simulink model "DuoCopter1AGRESSIVE"  (R2015b)
settings: Solver=FixedStepAuto  StartTime=0.0  StopTime=100  FixedStep=.01  MaxStep=10  RelTol=1e-3
values from neighbouring files (symbols this model uses):
  AoAMax = 18    [MainDataFile.m]
  RodMass = 1505    [MainDataFile.m]
  s = saveObjectImpl@matlab.System(obj)    [moving_average.m]
undefined symbols (not defined in the file or in its folder): X, Y, Z
libraries: sm_lib x35, Library_Octocopter x19, nesl_utility x17, simulink x3, aerolibfltsims x2
(part 1 of 2)
settings Model: Creator=John  LastModifiedBy=hielke
settings SolverCC: AutoInsertRateTranBlk=on
settings DataIOCC: SaveFormat=Array
settings OptimizationCC: OptimizeBlockIOStorage=off  BufferReuse=off  GlobalBufferReuse=off  ExpressionFolding=off  LocalBlockOutputs=off
settings DebuggingCC: UnderspecifiedInitializationDetection=Classic  MergeDetectMultiDrivingBlocksExec=none  SolverPrmCheckMsg=warning
settings HardwareCC: ProdBitPerLong=64  ProdHWDeviceType=Intel->x86-64 (Linux 64)
settings GRTTargetCC: GeneratePreprocessorConditionals=Disable all
settings ConfigComp: CovModelRefEnable=Off

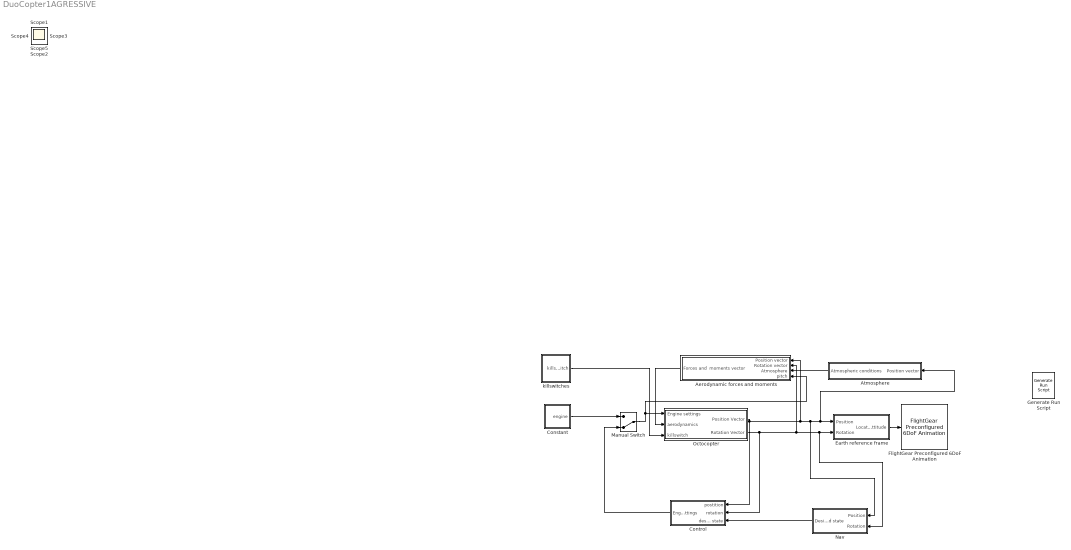
== system DuoCopter1AGRESSIVE ==
  Aerodynamic forces and moments : Subsystem
  Atmosphere : Subsystem
  Constant : Subsystem
  Control : Subsystem
  Earth reference frame : Subsystem
  FlightGear Preconfigured 6DoF Animation : aerolibfltsims/FlightGear Preconfigured 6DoF Animation  xFlightGearVersion=v3.4  DestinationIpAddress=127.0.0.1  DestinationPort=5502  SampleTime=-1
  Generate Run Script : aerolibfltsims/Generate Run Script  OutputFileName=runfg.sh  FlightGearBaseDirectory=/usr/share/games/flightgear  GeometryModelName=HL20  DestinationPort=5502  OriginAddress=127.0.0.1  OriginPort=5505  LocalAddress=127.0.0.1  AirportId=KSFO  RunwayId=10L  InitialAltitude=7224  InitialHeading=113  OffsetDistance=4.72  OffsetAzimuth=0  GenerateFile=off  Architecture=Linux  dataFlow=Send
  Manual Switch : ManualSwitch  CurrentSetting=0
  Nav : Subsystem
  Octocopter : Subsystem  SystemSampleTime=0.01
      settings: MinAlgLoopOccurrences=on
  killswitches : Subsystem
  Scope{,1..5} (6 alike) : Scope
  wires:
  Octocopter/2(Rotation Vector) -> Control/2(rotation), Aerodynamic forces and moments/2(Rotation vector), Nav/2(Rotation), Earth reference frame/2(Rotation)
  Octocopter/1(Position Vector) -> Control/1(postition), Aerodynamic forces and moments/1(Position vector), Nav/1(Position), Atmosphere/1(Position vector), Earth reference frame/1(Position)
  Nav/1(Desired state) -> Control/3(desired state)
  Earth reference frame/1(Location and attitude) -> FlightGear Preconfigured 6DoF Animation/1
  Control/1(Engine settings) -> Manual Switch/2
  Constant/1(engine) -> Manual Switch/1
  Manual Switch/1 -> Aerodynamic forces and moments/4(pitch), Octocopter/1(Engine settings)
  Aerodynamic forces and moments/1(Forces and  moments vector) -> Octocopter/2(aerodynamics)
  Atmosphere/1(Atmospheric conditions) -> Aerodynamic forces and moments/3(Atmosphere)
  killswitches/1(killswitch) -> Octocopter/3("killswitch ")

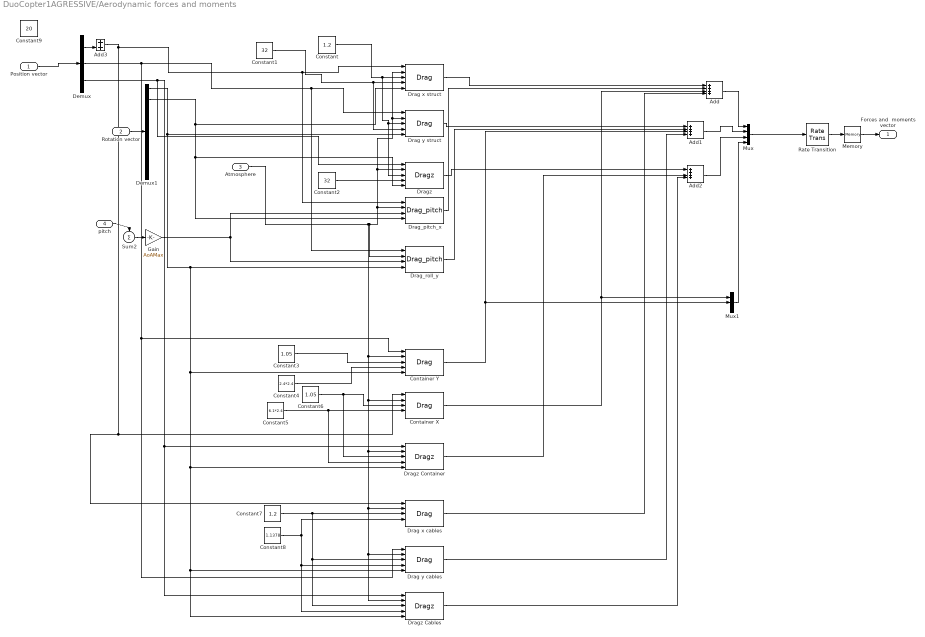
== system DuoCopter1AGRESSIVE/Aerodynamic forces and moments ==
  Position vector : Inport
  Rotation vector : Inport  Port=2
  Atmosphere : Inport  Port=3
  pitch : Inport  Port=4
  Add : Sum  Inputs=++++
  Add1 : Sum  Inputs=++++
  Add2 : Sum  Inputs=++++
  Add3 : Sum
  Constant : Constant  Value=1.2  SampleTime=1
  Constant1 : Constant  Value=32  SampleTime=1
  Constant2 : Constant  Value=32  SampleTime=1
  Constant3 : Constant  Value=1.05  SampleTime=1
  Constant4 : Constant  Value=2.4*2.4  SampleTime=1
  Constant5 : Constant  Value=6.1*2.4  SampleTime=1
  Constant6 : Constant  Value=1.05  SampleTime=1
  Constant7 : Constant  Value=1.2  SampleTime=1
  Constant8 : Constant  Value=1.1378  SampleTime=1
  Constant9 : Constant  Value=20
  Container X : Library_Octocopter/Drag
  Container Y : Library_Octocopter/Drag
  Demux : Demux  Outputs=9
  Demux1 : Demux  Outputs=9
  Drag x cables : Library_Octocopter/Drag
  Drag x struct : Library_Octocopter/Drag
  Drag y cables : Library_Octocopter/Drag
  Drag y struct : Library_Octocopter/Drag
  Drag_pitch_x : Library_Octocopter/Drag_pitch
  Drag_roll_y : Library_Octocopter/Drag_pitch
  "Dragz " : Library_Octocopter/Dragz 
  Dragz Cables : Library_Octocopter/Dragz 
  Dragz Container : Library_Octocopter/Dragz 
  Gain : Gain  Gain=AoAMax
  Memory : Memory  InheritSampleTime=on  LinearizeMemory=on  LinearizeAsDelay=on
  Mux : Mux
  Mux1 : Mux  Inputs=3
  Rate Transition : RateTransition  OutPortSampleTimeOpt=Inherit
  Sum2 : Sum  Inputs=+|
  Forces and  moments vector : Outport
  wires:
  Position vector/1 -> Demux/1
  Demux/5 -> Drag y cables/1, Container Y/1, Drag_roll_y/1, Drag y struct/1
  Atmosphere/1 -> Container X/2, Dragz Container/2, Drag x cables/2, Dragz Cables/2, Drag y cables/2, Container Y/2, Drag_roll_y/2, "Dragz "/2, Drag x struct/2, Drag y struct/2, Drag_pitch_x/2
  Constant/1 -> Drag x struct/3, "Dragz "/3, Drag y struct/3
  Constant1/1 -> Drag y struct/4, Drag x struct/4
  Constant2/1 -> "Dragz "/4
  Add3/1 -> Drag_pitch_x/1, Drag x struct/1, Drag x cables/1, Container X/1
  Demux/8 -> Dragz Cables/1, Dragz Container/1, "Dragz "/1
  Rotation vector/1 -> Demux1/1
  Demux1/1 -> Drag y struct/5, Dragz Cables/5, Drag y cables/5, Dragz Container/5, Container Y/5, Drag_roll_y/4
  Demux1/2 -> Drag x struct/5, "Dragz "/5, Drag_pitch_x/4
  Add1/1 -> Mux/2
  Drag x struct/1 -> Add/1
  Add/1 -> Mux/1
  Mux/1 -> Rate Transition/1
  pitch/1 -> Sum2/1
  Sum2/1 -> Gain/1
  Gain/1 -> Drag_roll_y/3, Drag_pitch_x/3
  Drag y struct/1 -> Add1/1
  Drag_roll_y/1 -> Add1/2
  Drag_pitch_x/1 -> Add/2
  Mux1/1 -> Mux/4
  Rate Transition/1 -> Memory/1
  Memory/1 -> Forces and  moments vector/1
  Constant3/1 -> Container Y/3
  Constant4/1 -> Container Y/4
  Constant5/1 -> Dragz Container/4, Container X/4
  Constant6/1 -> Dragz Container/3, Container X/3
  Constant7/1 -> Drag x cables/3, Dragz Cables/3, Drag y cables/3
  Constant8/1 -> Drag x cables/4, Dragz Cables/4, Drag y cables/4
  Container X/1 -> Add/3, Mux1/1
  Container Y/1 -> Mux1/2, Add1/3
  Drag x cables/1 -> Add/4
  Drag y cables/1 -> Add1/4
  "Dragz "/1 -> Add2/1
  Add2/1 -> Mux/3
  Dragz Container/1 -> Add2/3
  Dragz Cables/1 -> Add2/4
  Demux/2 -> Add3/2

== system DuoCopter1AGRESSIVE/Atmosphere ==
  Position vector : Inport
  Demux : Demux  Outputs=9
  MATLAB Function : MATLAB Function  TreatAsAtomicUnit=on  SystemSampleTime=10
      settings: MinAlgLoopOccurrences=on
  Rate Transition : RateTransition  X0=1.225  OutPortSampleTime=10
  Rate Transition1 : RateTransition  X0=1.225
  Atmospheric conditions : Outport
  wires:
  Position vector/1 -> Rate Transition/1
  Demux/3 -> MATLAB Function/1(u)
  MATLAB Function/1(y) -> Rate Transition1/1
  Rate Transition/1 -> Demux/1
  Rate Transition1/1 -> Atmospheric conditions/1

== system DuoCopter1AGRESSIVE/Constant ==
  Constant7 : Constant  Value=0.835
  Mux : Mux  Inputs=8
  engine : Outport
  wires:
  Mux/1 -> engine/1
  Constant7/1 -> Mux/1, Mux/2, Mux/3, Mux/4, Mux/5, Mux/6, Mux/7, Mux/8

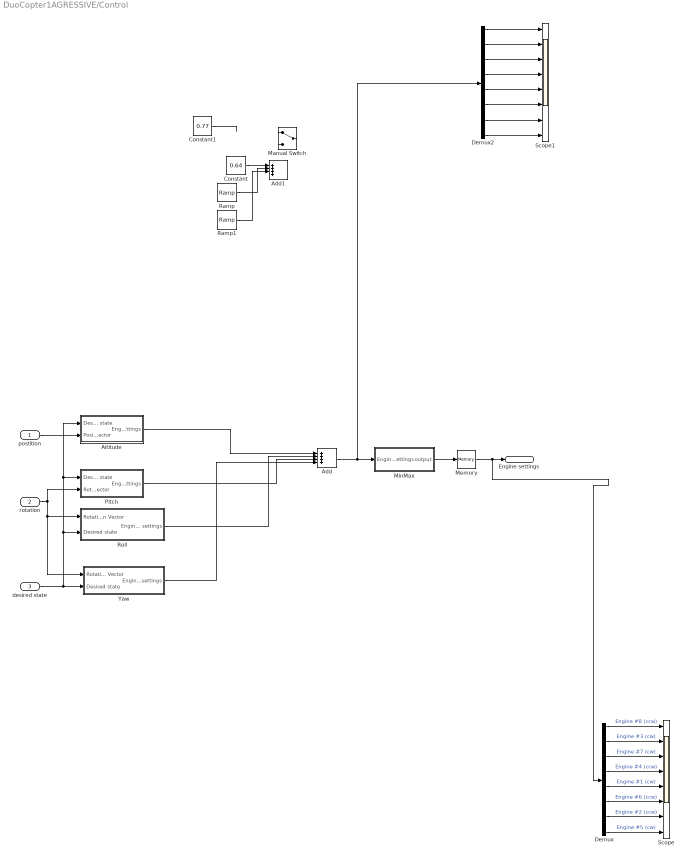
== system DuoCopter1AGRESSIVE/Control ==
  postition : Inport
  rotation : Inport  Port=2
  desired state : Inport  Port=3
  Add : Sum  Inputs=++++
  Add1 : Sum  Inputs=++++
  Altitude : Subsystem
  Constant : Constant  Value=0.64
  Constant1 : Constant  Value=0.77
  Demux : Demux  Outputs=8
  Demux2 : Demux  Outputs=8
  Manual Switch : ManualSwitch
  Memory : Memory  X0=0.84  InheritSampleTime=on  LinearizeMemory=on  LinearizeAsDelay=on
  MinMax : Subsystem
  Pitch : Subsystem
  Ramp : simulink/Sources/Ramp  slope=.014  start=20  X0=0
  Ramp1 : simulink/Sources/Ramp  slope=-.014  start=42  X0=0
  Roll : Subsystem
  Scope : Scope  NumInputPorts=8
  Scope1 : Scope  NumInputPorts=8
  Yaw : Subsystem
  Engine settings : Outport
  wires:
  Roll/1(Engine settings) -> Add/2
  Pitch/1(Engine settings) -> Add/3
  Yaw/1(Engine settings) -> Add/4
  Demux/1 -> Scope/1  "Engine #8 (ccw)"
  Demux/2 -> Scope/2  "Engine #3 (cw)"
  Demux/3 -> Scope/3  "Engine #7 (cw)"
  Demux/4 -> Scope/4  "Engine #4 (ccw)"
  Demux/5 -> Scope/5  "Engine #1 (cw)"
  Demux/6 -> Scope/6  "Engine #6 (ccw)"
  Demux/7 -> Scope/7  "Engine #2 (ccw)"
  Demux/8 -> Scope/8  "Engine #5 (cw)"
  Demux2/1 -> Scope1/1
  Demux2/2 -> Scope1/2
  Demux2/3 -> Scope1/3
  Demux2/4 -> Scope1/4
  Demux2/5 -> Scope1/5
  Demux2/6 -> Scope1/6
  Demux2/7 -> Scope1/7
  Demux2/8 -> Scope1/8
  Memory/1 -> Demux/1, Engine settings/1
  Add/1 -> Demux2/1, MinMax/1(Engine settings)
  rotation/1 -> Yaw/1(Rotation Vector), Roll/1(Rotation Vector), Pitch/2(Rotation Vector)
  desired state/1 -> Yaw/2(Desired state), Altitude/1(Desired state), Pitch/1(Desired state), Roll/2(Desired state)
  postition/1 -> Altitude/2(Position Vector)
  MinMax/1(output) -> Memory/1
  Constant/1 -> Add1/1
  Constant1/1 -> ?
  Ramp/1 -> Add1/2
  Ramp1/1 -> Add1/3
  Altitude/1(Engine settings) -> Add/1

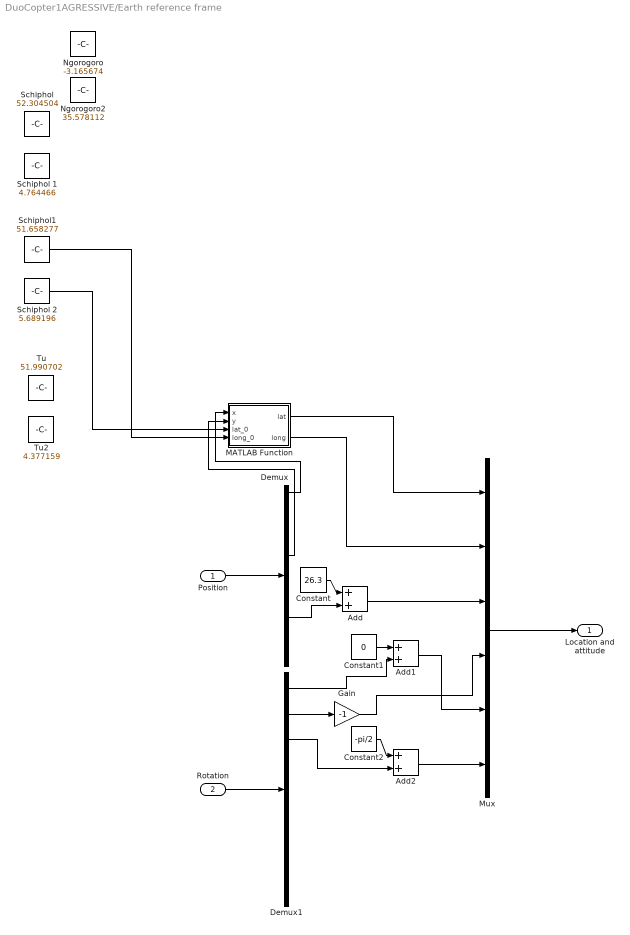
== system DuoCopter1AGRESSIVE/Earth reference frame ==
  Position : Inport
  Rotation : Inport  Port=2
  Add : Sum
  Add1 : Sum
  Add2 : Sum
  Constant : Constant  Value=26.3
  Constant1 : Constant  Value=0
  Constant2 : Constant  Value=-pi/2
  Demux : Demux  Outputs=9
  Demux1 : Demux  Outputs=9
  Gain : Gain  Gain=-1
  MATLAB Function : MATLAB Function  TreatAsAtomicUnit=on
  Mux : Mux  Inputs=6
  Ngorogoro : Constant  Value=-3.165674
  Ngorogoro2 : Constant  Value=35.578112
  Schiphol : Constant  Value=52.304504
  Schiphol 1 : Constant  Value=4.764466
  Schiphol 2 : Constant  Value=5.689196
  Schiphol1 : Constant  Value=51.658277
  Tu : Constant  Value=51.990702
  "Tu2 " : Constant  Value=4.377159
  Location and attitude : Outport
  wires:
  Position/1 -> Demux/1
  Rotation/1 -> Demux1/1
  Demux1/2 -> Gain/1
  Mux/1 -> Location and attitude/1
  Demux/7 -> Add/2
  Constant/1 -> Add/1
  Add/1 -> Mux/3
  Demux/1 -> MATLAB Function/1(x)
  Demux/4 -> MATLAB Function/2(y)
  MATLAB Function/1(lat) -> Mux/1
  MATLAB Function/2(long) -> Mux/2
  Demux1/1 -> Add1/2
  Constant1/1 -> Add1/1
  Add1/1 -> Mux/5
  Schiphol1/1 -> MATLAB Function/4(long_0)
  Schiphol 2/1 -> MATLAB Function/3(lat_0)
  Demux1/3 -> Add2/2
  Constant2/1 -> Add2/1
  Add2/1 -> Mux/6
  Gain/1 -> Mux/4

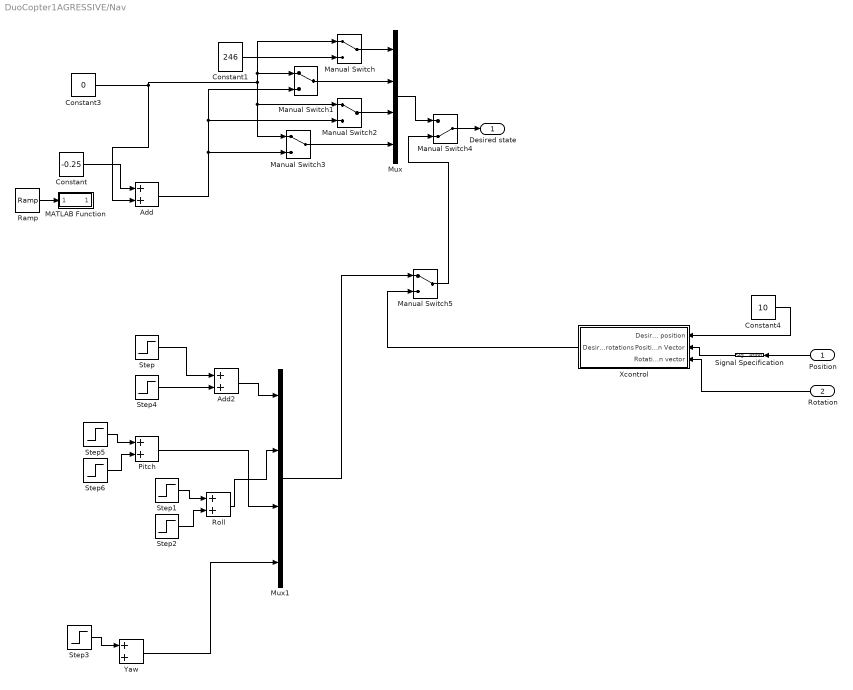
== system DuoCopter1AGRESSIVE/Nav ==
  Position : Inport
  Rotation : Inport  Port=2
  Add : Sum
  Add2 : Sum
  Constant : Constant  Value=-0.25
  Constant1 : Constant  Value=246
  Constant3 : Constant  Value=0
  Constant4 : Constant  Value=10
  MATLAB Function : MATLAB Function  TreatAsAtomicUnit=on
  Manual Switch{,1..3,5} (5 alike) : ManualSwitch
  Manual Switch4 : ManualSwitch  CurrentSetting=0
  Mux : Mux
  Mux1 : Mux
  Pitch : Sum
  Ramp : simulink/Sources/Ramp  slope=-0.025  start=0  X0=0.5
  Roll : Sum
  Signal Specification : SignalSpecification  Dimensions=9
  Step : Step  Time=5  After=25
  Step1 : Step  Time=42  After=-0.3
  Step2 : Step  Time=50  After=0.3
  Step3 : Step  Time=42  After=-0.4
  Step4 : Step  Time=28  After=200
  Step5 : Step  Time=15  After=0.3
  Step6 : Step  Time=25  After=-0.1
  Xcontrol : Subsystem
  Yaw : Sum
  Desired state : Outport
  wires:
  Manual Switch/1 -> Mux/1
  Manual Switch1/1 -> Mux/2
  Manual Switch2/1 -> Mux/3
  Manual Switch3/1 -> Mux/4
  Constant3/1 -> Manual Switch3/1, Manual Switch2/1, Manual Switch/1, Manual Switch1/1, Add/2
  Constant/1 -> Add/1
  Constant1/1 -> Manual Switch/2
  Ramp/1 -> MATLAB Function/1(input)
  Add/1 -> Manual Switch3/2, Manual Switch2/2, Manual Switch1/2
  Manual Switch4/1 -> Desired state/1
  Mux/1 -> Manual Switch4/1
  Position/1 -> Signal Specification/1
  Manual Switch5/1 -> Manual Switch4/2
  Mux1/1 -> Manual Switch5/1
  Xcontrol/1(Desired rotations) -> Manual Switch5/2
  Constant4/1 -> Xcontrol/1(Desired position)
  Signal Specification/1 -> Xcontrol/2(Position Vector)
  Rotation/1 -> Xcontrol/3(Rotation vector)
  Pitch/1 -> Mux1/3
  Add2/1 -> Mux1/1
  Step/1 -> Add2/1
  Step4/1 -> Add2/2
  Step2/1 -> Roll/2
  Step1/1 -> Roll/1
  Roll/1 -> Mux1/2
  Step6/1 -> Pitch/2
  Step5/1 -> Pitch/1
  Step3/1 -> Yaw/1
  Yaw/1 -> Mux1/4

== system DuoCopter1AGRESSIVE/Octocopter ==
  Engine settings : Inport
  aerodynamics : Inport  Port=2
  "killswitch " : Inport  Port=3
  6 DOF joint : Subsystem
  Demux : Demux  Outputs=8
  Horizontal 1 : Subsystem
  Horizontal 2 : Subsystem
  Mechanism Configuration : sm_lib/Utilities/Mechanism Configuration  UniformGravity=Constant  GravityVector=[0 0 -9.81]  GravityUnits=m/s^2  LinearizationDelta=0.001  BlockFunction=simmechanics.library.utilities.mechanism_configuration
  Rigid Transform : sm_lib/Frames and Transforms/Rigid Transform  TranslationMethod=Cartesian  TranslationLengthUnit=m  TranslationStandardAxis=+Z  TranslationStandardOffset=0  TranslationCartesianOffset=[0 0 -1.3]  TranslationROffset=0  TranslationROffsetUnits=m  TranslationZOffset=0  TranslationZOffsetUnits=m  TranslationThetaOffset=0  TranslationThetaOffsetUnits=deg  RotationMethod=None  RotationAngleUnits=deg  RotationStandardAxis=+Z  RotationAngle=0.0  RotationArbitraryAxis=[0 0 1]  FollAlignAxisA=+X  BaseAlignAxisA=+Y  FollAlignAxisB=+Y  BaseAlignAxisB=+Z  RotationSequenceAxes=FollowerAxes  RotationSequence=XYX  RotationSequenceAngles=[0 0 0]  RotationSequenceAnglesUnits=deg  RotationMatrix=[1 0 0; 0 1 0; 0 0 1]  BlockFunction=simmechanics.library.frames_transforms.rigid_transform
  Solid : sm_lib/Body Elements/Solid  InertiaType=CalculateFromGeometry  Mass=5000  MassUnits=kg  CenterOfMass=[0 0 0]  CenterOfMassUnits=m  MomentsOfInertia=[1 1 1]  MomentsOfInertiaUnits=kg*m^2  ProductsOfInertia=[0 0 0]  ProductsOfInertiaUnits=kg*m^2  DensityBased=on  Density=128.205  DensityUnits=kg/(m^3)  DoExposeReferenceFrame=on  SerializedFrames=<Frames/>  GraphicType=FromGeometry  MarkerShape=Sphere  MarkerSize=10  MarkerSizeUnits=m  GraphicVisPropType=SimpleVisualProperties  GraphicDiffuseColor=[0.5 0.5 0.5]  GraphicSpecularColor=[0.5 0.5 0.5 1.0]  GraphicAmbientColor=[0.15 0.15 0.15 1.0]  GraphicEmissiveColor=[0.0 0.0 0.0 1.0]  GraphicShininess=75  GraphicOpacity=1.0  GeometryShape=Brick  RectangleSize=[1 1]  RectangleSizeUnits=m  BrickDimensions=[2.44 6.1 2.59]  BrickDimensionUnits=m  CylinderRadius=1  CylinderRadiusUnits=m  CylinderLength=1  CylinderLengthUnits=m  SphereRadius=1  SphereRadiusUnits=m  EllipsoidRadii=[1 1 1]  EllipsoidRadiiUnits=m  ExtrusionCrossSection=[1 1; -1 1; -1 -1; 1 -1]  ExtrusionCrossSectionUnits=m  ExtrusionLength=1  ExtrusionLengthUnits=m  PolygonNumSides=3  PolygonOuterRadius=1  PolygonOuterRadiusUnits=m  ExtGeomFileType=STL  ExtGeomFileUnits=m  RevolutionCrossSection=[1 1; 1 -1; 2 -1; 2 1]  RevolutionCrossSectionUnits=m  RevolutionExtent=Full  RevolutionAngle=180  RevolutionAngleUnits=deg  BlockFunction=simmechanics.library.body_elements.solid
  Solver Configuration : nesl_utility/Solver Configuration  PhysicalDomain=network_engine_domain  SubClassName=solver  LeftPortType=input  RightPortType=generic  Accelerate=off  Tones=[]  Harmonics=[]  SimulateNoise=off  Profile=off  UseLocalSampling=off  EnableSwitchedLinearOptims=on  FrequencyDomain=off  UseCCode=off  RelTol=0.001  AbsTol=1e-06  MinStep=1e-09  ToWorkspace=off  RevertToSquareIcSolve=off  NumHomotopyIterations=100  PhasorMode=off  PhasorModeNumHarmonics=1  DoDC=off  ResidualTolerance=1e-09  UseLocalSolver=off  LocalSolverChoice=NE_BACKWARD_EULER_ADVANCER  LocalSolverSampleTime=0.001  DoFixedCost=off  MaxNonlinIter=3  MaxModeIter=2  LinearAlgebra=Sparse  DelaysMemoryBudget=1024  AutomaticFiltering=on  FilteringTimeConstant=0.001
  Vertical 1 : Subsystem
  Vertical 2 : Subsystem
  World Frame : sm_lib/Frames and Transforms/World Frame  BlockFunction=simmechanics.library.frames_transforms.world_frame
  Position Vector : Outport
  Rotation Vector : Outport  Port=2
  wires:
  Demux/6 -> Vertical 1/2(Motor 6 ccw)
  Demux/8 -> Vertical 2/2(Motor 5 cw)
  6 DOF joint/2(Rotation Vector) -> Rotation Vector/1
  6 DOF joint/1(Position Vector) -> Position Vector/1
  Demux/5 -> Vertical 1/1(Motor 1 cw)
  Demux/1 -> Horizontal 1/1(Motor 8 ccw)
  Demux/7 -> Vertical 2/1("Motor 2 ccw ")
  Demux/4 -> Horizontal 2/2(Motor 4 ccw)
  Demux/2 -> Horizontal 1/2(Motor 3 cw)
  Engine settings/1 -> Demux/1
  Demux/3 -> Horizontal 2/1(Motor 7 cw)
  aerodynamics/1 -> 6 DOF joint/1("aerodynamic forces and moment ")
  connections:
  Horizontal 1/RConn1 -- Rigid Transform/LConn1 -- Vertical 2/RConn1 -- Vertical 1/RConn1 -- 6 DOF joint/LConn1 -- Horizontal 2/RConn1
  Solver Configuration/RConn1 -- Mechanism Configuration/RConn1 -- 6 DOF joint/LConn2 -- World Frame/RConn1
  Solid/RConn1 -- Rigid Transform/RConn1

== system DuoCopter1AGRESSIVE/killswitches ==
  Constant : Constant  Value=0  SampleTime=1
  Constant1 : Constant  SampleTime=1
  Manual Switch{,1..6} (7 alike) : ManualSwitch
  Manual Switch7 : ManualSwitch  CurrentSetting=0
  Mux : Mux  Inputs=8
  killswitch : Outport
  wires:
  Constant/1 -> Manual Switch2/1, Manual Switch1/1, Manual Switch/1, Manual Switch5/1, Manual Switch6/1, Manual Switch7/1, Manual Switch4/1, Manual Switch3/1
  Constant1/1 -> Manual Switch4/2, Manual Switch3/2, Manual Switch2/2, Manual Switch1/2, Manual Switch/2, Manual Switch7/2, Manual Switch6/2, Manual Switch5/2
  Manual Switch7/1 -> Mux/8
  Manual Switch6/1 -> Mux/7
  Manual Switch5/1 -> Mux/6
  Manual Switch4/1 -> Mux/5
  Manual Switch3/1 -> Mux/4
  Manual Switch2/1 -> Mux/3
  Manual Switch1/1 -> Mux/2
  Manual Switch/1 -> Mux/1
  Mux/1 -> killswitch/1

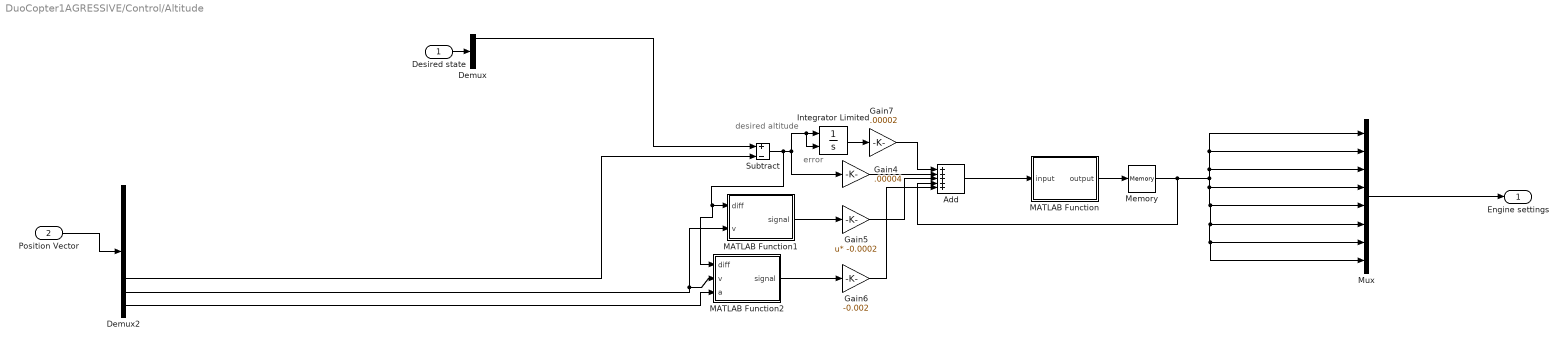
== system DuoCopter1AGRESSIVE/Control/Altitude ==
  note: error
  note: desired altitude
  Desired state : Inport
  Position Vector : Inport  Port=2
  Add : Sum  Inputs=+++++
  Demux : Demux
  Demux2 : Demux  Outputs=9
  Gain4 : Gain  Gain=.00004
  Gain5 : Gain  Gain=-0.0002  Multiplication=Matrix(u*K)
  Gain6 : Gain  Gain=-0.002
  Gain7 : Gain  Gain=.00002
  Integrator Limited : Integrator  ExternalReset=either  LimitOutput=on  UpperSaturationLimit=100  LowerSaturationLimit=-100
  MATLAB Function : MATLAB Function  TreatAsAtomicUnit=on
  MATLAB Function1 : MATLAB Function  TreatAsAtomicUnit=on
  MATLAB Function2 : MATLAB Function  TreatAsAtomicUnit=on
  Memory : Memory  X0=0.7  LinearizeAsDelay=on
  Mux : Mux  Inputs=8
  Subtract : Sum  Inputs=+-
  Engine settings : Outport
  wires:
  Position Vector/1 -> Demux2/1
  Desired state/1 -> Demux/1
  Integrator Limited/1 -> Gain7/1
  Subtract/1 -> MATLAB Function2/1(diff), MATLAB Function1/1(diff), Integrator Limited/2, Integrator Limited/1, Gain4/1
  Demux2/9 -> MATLAB Function2/3(a)
  Gain7/1 -> Add/1
  Gain5/1 -> Add/3
  Add/1 -> MATLAB Function/1(input)
  MATLAB Function/1(output) -> Memory/1
  Gain4/1 -> Add/2
  Demux/1 -> Subtract/1
  Demux2/7 -> Subtract/2
  Mux/1 -> Engine settings/1
  Memory/1 -> Add/4, Mux/8, Mux/7, Mux/6, Mux/5, Mux/4, Mux/1, Mux/2, Mux/3
  Gain6/1 -> Add/5
  Demux2/8 -> MATLAB Function2/2(v), MATLAB Function1/2(v)
  MATLAB Function1/1(signal) -> Gain5/1
  MATLAB Function2/1(signal) -> Gain6/1

== system DuoCopter1AGRESSIVE/Control/MinMax ==
  Engine settings : Inport
  Demux1 : Demux  Outputs=8
  MATLAB Function : MATLAB Function  TreatAsAtomicUnit=on
  MATLAB Function1 : MATLAB Function  TreatAsAtomicUnit=on
  MATLAB Function2 : MATLAB Function  TreatAsAtomicUnit=on
  MATLAB Function3 : MATLAB Function  TreatAsAtomicUnit=on
  MATLAB Function4 : MATLAB Function  TreatAsAtomicUnit=on
  MATLAB Function5 : MATLAB Function  TreatAsAtomicUnit=on
  MATLAB Function6 : MATLAB Function  TreatAsAtomicUnit=on
  MATLAB Function7 : MATLAB Function  TreatAsAtomicUnit=on
  Mux : Mux  Inputs=8
  Signal Specification : SignalSpecification  Dimensions=8
  output : Outport
  wires:
  Demux1/6 -> MATLAB Function5/1(input)
  Demux1/7 -> MATLAB Function6/1(input)
  MATLAB Function6/1(output) -> Mux/7
  Engine settings/1 -> Signal Specification/1
  Signal Specification/1 -> Demux1/1
  MATLAB Function5/1(output) -> Mux/6
  MATLAB Function7/1(output) -> Mux/8
  Demux1/2 -> MATLAB Function1/1(input)
  Demux1/3 -> MATLAB Function2/1(input)
  Demux1/4 -> MATLAB Function3/1(input)
  Mux/1 -> output/1
  Demux1/1 -> MATLAB Function/1(input)
  MATLAB Function4/1(output) -> Mux/5
  MATLAB Function3/1(output) -> Mux/4
  Demux1/5 -> MATLAB Function4/1(input)
  MATLAB Function/1(output) -> Mux/1
  MATLAB Function1/1(output) -> Mux/2
  MATLAB Function2/1(output) -> Mux/3
  Demux1/8 -> MATLAB Function7/1(input)

== system DuoCopter1AGRESSIVE/Control/Pitch ==
  Desired state : Inport
  Rotation Vector : Inport  Port=2
  Demux : Demux
  Demux2 : Demux  Outputs=9
  Pitchsub : Subsystem
  Engine settings : Outport
  wires:
  Rotation Vector/1 -> Demux2/1
  Pitchsub/1(Engine settings) -> Engine settings/1
  Demux2/1 -> Pitchsub/2(theta)
  Demux2/4 -> Pitchsub/3(theta_d)
  Demux2/7 -> Pitchsub/4(theta_dd)
  Desired state/1 -> Demux/1
  Demux/3 -> Pitchsub/1(desired pitch)

== system DuoCopter1AGRESSIVE/Control/Roll ==
  Rotation Vector : Inport
  Desired state : Inport  Port=2
  Demux : Demux
  Demux2 : Demux  Outputs=9
  Rollsub : Subsystem
  Scope : Scope  NumInputPorts=3
  Engine settings : Outport
  wires:
  Rotation Vector/1 -> Demux2/1
  Rollsub/1(Engine settings) -> Engine settings/1
  Demux2/2 -> Scope/1, Rollsub/2(phi)  "Roll"
  Demux2/5 -> Rollsub/3(phi_d)
  Demux2/8 -> Rollsub/4(phi_dd)
  Desired state/1 -> Demux/1
  Demux2/1 -> Scope/2  "Pitch"
  Demux2/3 -> Scope/3  "Yaw"
  Demux/2 -> Rollsub/1(desired roll)

== system DuoCopter1AGRESSIVE/Control/Yaw ==
  Rotation Vector : Inport
  Desired state : Inport  Port=2
  Demux : Demux
  Demux2 : Demux  Outputs=9
  Yawsub : Subsystem
  Engine settings : Outport
  wires:
  Rotation Vector/1 -> Demux2/1
  Demux/4 -> Yawsub/1(desired heading)
  Demux2/3 -> Yawsub/2(psi)
  Demux2/6 -> Yawsub/3(psi_d)
  Demux2/9 -> Yawsub/4(psi_dd)
  Yawsub/1(Engine settings) -> Engine settings/1
  Desired state/1 -> Demux/1

== system DuoCopter1AGRESSIVE/Nav/Xcontrol ==
  Desired position : Inport
  Position Vector : Inport  Port=2
  Rotation vector : Inport  Port=3
  Constant : Constant  Value=0
  Demux : Demux  Outputs=9
  Demux2 : Demux  Outputs=9
  Mux : Mux
  Ycontrol : Subsystem
  Desired rotations : Outport
  wires:
  Position Vector/1 -> Demux2/1
  Desired position/1 -> Ycontrol/1(desired position)
  Mux/1 -> Desired rotations/1
  Ycontrol/1(pitch settings) -> Mux/3
  Demux2/5 -> Ycontrol/3(dy)
  Demux2/6 -> Ycontrol/4(ddy)
  Constant/1 -> Mux/2, Mux/4, Mux/1
  Demux2/4 -> Ycontrol/2(y)
  Rotation vector/1 -> Demux/1
  Demux/2 -> Ycontrol/5(theta)
  Demux/5 -> Ycontrol/6(d_theta)

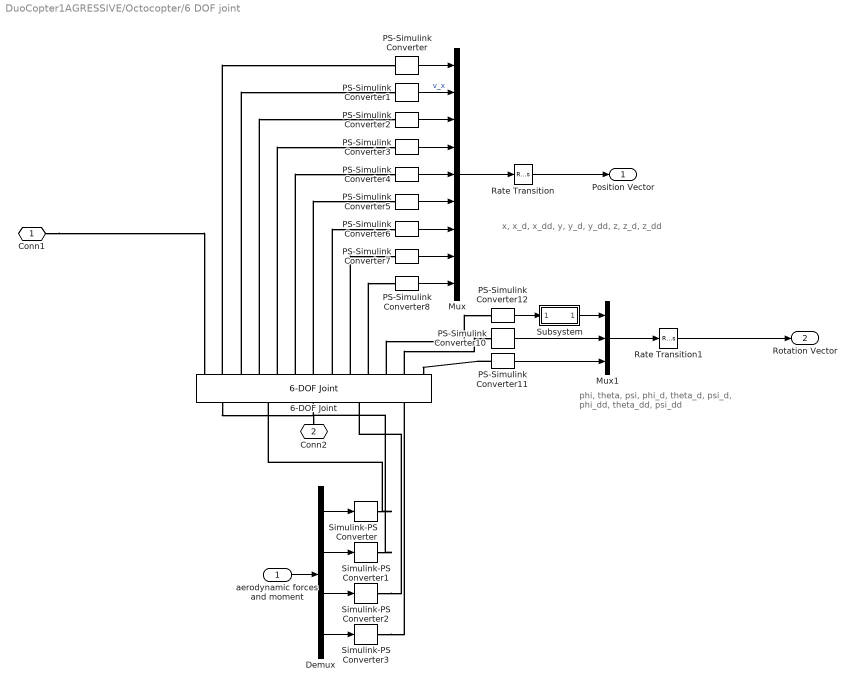
== system DuoCopter1AGRESSIVE/Octocopter/6 DOF joint ==
  note: x, x_d, x_dd, y, y_d, y_dd, z, z_d, z_dd
  note: phi, theta, psi, phi_d, theta_d, psi_d, phi_dd, theta_dd, psi_dd
  "aerodynamic forces and moment " : Inport
  6-DOF Joint : sm_lib/Joints/6-DOF Joint  SenseConstraintForce=off  SenseConstraintForceX=off  SenseConstraintForceY=off  SenseConstraintForceZ=off  SenseConstraintTorque=off  SenseConstraintTorqueX=off  SenseConstraintTorqueY=off  SenseConstraintTorqueZ=off  SenseTotalForce=off  SenseTotalForceX=off  SenseTotalForceY=off  SenseTotalForceZ=off  SenseTotalTorque=off  SenseTotalTorqueX=off  SenseTotalTorqueY=off  SenseTotalTorqueZ=off  CompositeWrenchDir=FollowerOnBase  CompositeWrenchFrame=BaseFrame  PxEquilibriumPosition=0  PxEquilibriumPositionUnits=m  PxSpringStiffness=0  PxSpringStiffnessUnits=N/m  PxDampingCoefficient=0  PxDampingCoefficientUnits=N/(m/s)  PxTorqueActuationMode=InputTorque  PxMotionActuationMode=ComputedMotion  PxSensePosition=on  PxSenseVelocity=on  PxSenseAcceleration=on  PxSenseTorqueForce=off  PxPositionTargetSpecify=off  PxPositionTargetPriority=High  PxPositionTargetValue=0  PxPositionTargetValueUnits=m  PxVelocityTargetSpecify=off  PxVelocityTargetPriority=High  PxVelocityTargetValue=0  PxVelocityTargetValueUnits=m/s  PyEquilibriumPosition=0  PyEquilibriumPositionUnits=m  PySpringStiffness=0  PySpringStiffnessUnits=N/m  PyDampingCoefficient=0  PyDampingCoefficientUnits=N/(m/s)  PyTorqueActuationMode=InputTorque  PyMotionActuationMode=ComputedMotion  PySensePosition=on  PySenseVelocity=on  PySenseAcceleration=on  PySenseTorqueForce=off  PyPositionTargetSpecify=off  PyPositionTargetPriority=High  PyPositionTargetValue=0  PyPositionTargetValueUnits=m  PyVelocityTargetSpecify=off  PyVelocityTargetPriority=High  PyVelocityTargetValue=0  PyVelocityTargetValueUnits=m/s  PzEquilibriumPosition=0  PzEquilibriumPositionUnits=m  PzSpringStiffness=0  PzSpringStiffnessUnits=N/m  PzDampingCoefficient=0  PzDampingCoefficientUnits=N/(m/s)  PzTorqueActuationMode=InputTorque  PzMotionActuationMode=ComputedMotion  PzSensePosition=on  PzSenseVelocity=on  PzSenseAcceleration=on  PzSenseTorqueForce=off  PzPositionTargetSpecify=off  PzPositionTargetPriority=High  PzPositionTargetValue=0  PzPositionTargetValueUnits=m  PzVelocityTargetSpecify=off  PzVelocityTargetPriority=High  PzVelocityTargetValue=0  PzVelocityTargetValueUnits=m/s  SphDefPosRotationMethod=None  SphDefPosRotationAngleUnits=deg  SphDefPosRotationStandardAxis=+Z  SphDefPosRotationAngle=0  SphDefPosRotationArbitraryAxis=[0 0 1]  SphDefPosFollAlignAxisA=+X  SphDefPosBaseAlignAxisA=+Y  SphDefPosFollAlignAxisB=+Y  SphDefPosBaseAlignAxisB=+Z  SphDefPosRotationSequenceAxes=FollowerAxes  SphDefPosRotationSequence=XYX  SphDefPosRotationSequenceAngles=[0 0 0]  SphDefPosRotationSequenceAnglesUnits=deg  SphDefPosRotationMatrix=[1 0 0; 0 1 0; 0 0 1]  SphEqPosRotationMethod=None  SphEqPosRotationAngleUnits=deg  SphEqPosRotationStandardAxis=+Z  SphEqPosRotationAngle=0  SphEqPosRotationArbitraryAxis=[0 0 1]  SphEqPosFollAlignAxisA=+X  SphEqPosBaseAlignAxisA=+Y  SphEqPosFollAlignAxisB=+Y  SphEqPosBaseAlignAxisB=+Z  SphEqPosRotationSequenceAxes=FollowerAxes  SphEqPosRotationSequence=XYX  SphEqPosRotationSequenceAngles=[0 0 0]  SphEqPosRotationSequenceAnglesUnits=deg  SphEqPosRotationMatrix=[1 0 0; 0 1 0; 0 0 1]  SphSpringStiffness=0  SphSpringStiffnessUnits=N*m/deg  SphDampingCoefficient=0  SphDampingCoefficientUnits=N*m/(deg/s)  SphActuateTorqueX=off  SphActuateTorqueY=off  SphActuateTorqueZ=off  SphActuateTorque=on  SphTorqueActuationMode=InputTorque  SphMotionActuationMode=ComputedMotion  SphActuationFrame=FollowerFrame  SphSensePosition=on  SphSenseVelocityX=off  SphSenseVelocityY=off  SphSenseVelocityZ=off  SphSenseVelocity=on  SphSenseAccelerationX=off  SphSenseAccelerationY=off  SphSenseAccelerationZ=off  SphSenseAcceleration=on  SphSenseTorqueX=off  SphSenseTorqueY=off  SphSenseTorqueZ=off  SphSenseTorqueForce=off  SphSensingFrame=BaseFrame  SphPositionTargetRotationMethod=None  SphPositionTargetRotationAngleUnits=deg  SphPositionTargetRotationStandardAxis=+Z  SphPositionTargetRotationAngle=0  SphPositionTargetRotationArbitraryAxis=[0 0 1]  SphPositionTargetFollAlignAxisA=+X  SphPositionTargetBaseAlignAxisA=+Y  SphPositionTargetFollAlignAxisB=+Y  SphPositionTargetBaseAlignAxisB=+Z  SphPositionTargetRotationSequenceAxes=FollowerAxes  SphPositionTargetRotationSequence=XYX  SphPositionTargetRotationSequenceAngles=[0 0 0]  SphPositionTargetRotationSequenceAnglesUnits=deg  SphPositionTargetRotationMatrix=[1 0 0; 0 1 0; 0 0 1]  SphPositionTargetSpecify=off  SphPositionTargetPriority=High  SphVelocityTargetValue=[0 0 0]  SphVelocityTargetValueUnits=deg/s  SphVelocityTargetSpecify=off  SphVelocityTargetPriority=High  SphVelocityTargetInFollowerFrame=on  BlockFunction=simmechanics.library.joints.sixdof_joint
  Demux : Demux
  Mux : Mux  Inputs=9
  Mux1 : Mux  Inputs=3
  PS-Simulink Converter{,1..5,8,11} (8 alike) : nesl_utility/PS-Simulink Converter  PhysicalDomain=network_engine_domain  SubClassName=ps_output  LeftPortType=input  RightPortType=output  PseudoPeriodic=off  Frequencies=[]  Unit=1  AffineConversion=off
  PS-Simulink Converter10 : nesl_utility/PS-Simulink Converter  PhysicalDomain=network_engine_domain  SubClassName=ps_output  LeftPortType=input  RightPortType=output  PseudoPeriodic=off  Frequencies=[]  Unit=rad/s  AffineConversion=off
  PS-Simulink Converter12 : nesl_utility/PS-Simulink Converter  PhysicalDomain=network_engine_domain  SubClassName=ps_output  LeftPortType=input  RightPortType=output  PseudoPeriodic=off  Frequencies=[]  Unit=rad  AffineConversion=off
  PS-Simulink Converter6 : nesl_utility/PS-Simulink Converter  PhysicalDomain=network_engine_domain  SubClassName=ps_output  LeftPortType=input  RightPortType=output  PseudoPeriodic=off  Frequencies=[]  Unit=m  AffineConversion=off
  PS-Simulink Converter7 : nesl_utility/PS-Simulink Converter  PhysicalDomain=network_engine_domain  SubClassName=ps_output  LeftPortType=input  RightPortType=output  PseudoPeriodic=off  Frequencies=[]  Unit=m/s  AffineConversion=off
  Rate Transition : RateTransition
  Rate Transition1 : RateTransition
  Simulink-PS Converter{,1..3} (4 alike) : nesl_utility/Simulink-PS Converter  PhysicalDomain=network_engine_domain  SubClassName=ps_input  LeftPortType=input  RightPortType=output  PseudoPeriodic=off  Frequencies=[]  NoiseDistribution=none  NoiseParameters=[]  Unit=1  AffineConversion=off  InputFiltering=off  SimscapeFilterOrder=1  InputFilterTimeConstant=0.001  UdotUserProvided=1
  Subsystem : Subsystem
  Conn1 : PMIOPort  Port=1  Side=Left
  Conn2 : PMIOPort  Port=2  Side=Left
  Position Vector : Outport
  Rotation Vector : Outport  Port=2
  wires:
  PS-Simulink Converter12/1 -> Subsystem/1(In1)
  PS-Simulink Converter/1 -> Mux/1
  PS-Simulink Converter1/1 -> Mux/2  "v_x"
  PS-Simulink Converter2/1 -> Mux/3
  PS-Simulink Converter3/1 -> Mux/4
  PS-Simulink Converter5/1 -> Mux/6
  PS-Simulink Converter6/1 -> Mux/7
  PS-Simulink Converter8/1 -> Mux/9
  PS-Simulink Converter7/1 -> Mux/8
  PS-Simulink Converter4/1 -> Mux/5
  Mux1/1 -> Rate Transition1/1
  Mux/1 -> Rate Transition/1
  Subsystem/1(Out1) -> Mux1/1
  PS-Simulink Converter10/1 -> Mux1/2
  PS-Simulink Converter11/1 -> Mux1/3
  Rate Transition/1 -> Position Vector/1
  Rate Transition1/1 -> Rotation Vector/1
  Demux/1 -> Simulink-PS Converter/1
  Demux/2 -> Simulink-PS Converter1/1
  Demux/3 -> Simulink-PS Converter2/1
  Demux/4 -> Simulink-PS Converter3/1
  "aerodynamic forces and moment "/1 -> Demux/1
  connections:
  6-DOF Joint/RConn4 -- PS-Simulink Converter2/LConn1
  6-DOF Joint/RConn12 -- PS-Simulink Converter10/LConn1
  6-DOF Joint/RConn11 -- PS-Simulink Converter12/LConn1
  6-DOF Joint/RConn3 -- PS-Simulink Converter1/LConn1
  6-DOF Joint/RConn10 -- PS-Simulink Converter8/LConn1
  6-DOF Joint/RConn6 -- PS-Simulink Converter4/LConn1
  PS-Simulink Converter11/LConn1 -- 6-DOF Joint/RConn13
  6-DOF Joint/RConn2 -- PS-Simulink Converter/LConn1
  6-DOF Joint/RConn8 -- PS-Simulink Converter6/LConn1
  6-DOF Joint/RConn5 -- PS-Simulink Converter3/LConn1
  6-DOF Joint/RConn9 -- PS-Simulink Converter7/LConn1
  6-DOF Joint/LConn1 -- Conn2/RConn1
  6-DOF Joint/RConn7 -- PS-Simulink Converter5/LConn1
  Conn1/RConn1 -- 6-DOF Joint/RConn1
  Simulink-PS Converter/RConn1 -- 6-DOF Joint/LConn2
  Simulink-PS Converter1/RConn1 -- 6-DOF Joint/LConn3
  Simulink-PS Converter2/RConn1 -- 6-DOF Joint/LConn4
  Simulink-PS Converter3/RConn1 -- 6-DOF Joint/LConn5

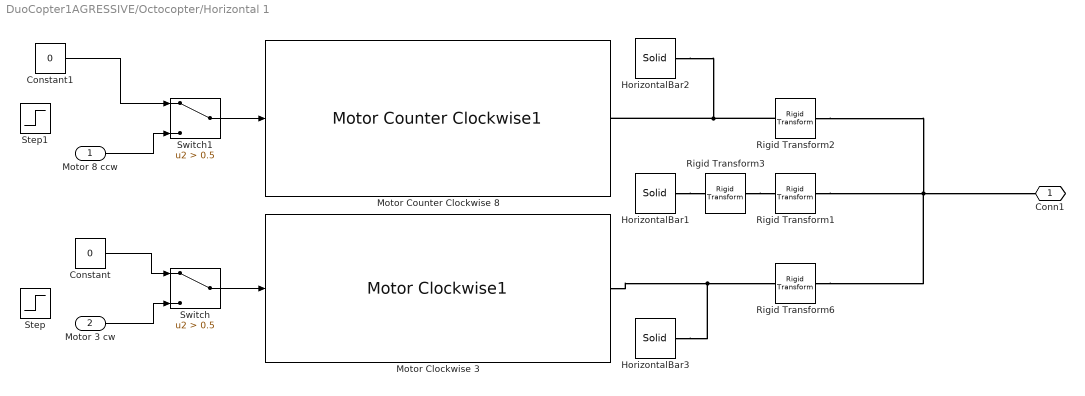
== system DuoCopter1AGRESSIVE/Octocopter/Horizontal 1 ==
  Motor 8 ccw : Inport
  Motor 3 cw : Inport  Port=2
  Constant : Constant  Value=0
  Constant1 : Constant  Value=0
  HorizontalBar1 : sm_lib/Body Elements/Solid  InertiaType=CalculateFromGeometry  Mass=RodMass  MassUnits=kg  CenterOfMass=[0 0 0]  CenterOfMassUnits=m  MomentsOfInertia=[1 1 1]  MomentsOfInertiaUnits=kg*m^2  ProductsOfInertia=[0 0 0]  ProductsOfInertiaUnits=kg*m^2  DensityBased=off  Density=DensityTube  DensityUnits=kg/(m^3)  DoExposeReferenceFrame=on  SerializedFrames=<Frames/>  GraphicType=FromGeometry  MarkerShape=Sphere  MarkerSize=10  MarkerSizeUnits=m  GraphicVisPropType=SimpleVisualProperties  GraphicDiffuseColor=[0.5 0.5 0.5]  GraphicSpecularColor=[0.5 0.5 0.5 1.0]  GraphicAmbientColor=[0.15 0.15 0.15 1.0]  GraphicEmissiveColor=[0.0 0.0 0.0 1.0]  GraphicShininess=75  GraphicOpacity=1.0  GeometryShape=Cylinder  RectangleSize=[1 1]  RectangleSizeUnits=m  BrickDimensions=[1 1 1]  BrickDimensionUnits=m  CylinderRadius=RadiusTube  CylinderRadiusUnits=m  CylinderLength=RodLength  CylinderLengthUnits=m  SphereRadius=1  SphereRadiusUnits=m  EllipsoidRadii=[1 1 1]  EllipsoidRadiiUnits=m  ExtrusionCrossSection=[1 1; -1 1; -1 -1; 1 -1]  ExtrusionCrossSectionUnits=m  ExtrusionLength=1  ExtrusionLengthUnits=m  PolygonNumSides=3  PolygonOuterRadius=1  PolygonOuterRadiusUnits=m  ExtGeomFileType=STL  ExtGeomFileUnits=m  RevolutionCrossSection=[1 1; 1 -1; 2 -1; 2 1]  RevolutionCrossSectionUnits=m  RevolutionExtent=Full  RevolutionAngle=180  RevolutionAngleUnits=deg  BlockFunction=simmechanics.library.body_elements.solid
  HorizontalBar2 : sm_lib/Body Elements/Solid  InertiaType=PointMass  Mass=462.5  MassUnits=kg  CenterOfMass=[0 0 0]  CenterOfMassUnits=m  MomentsOfInertia=[1 1 1]  MomentsOfInertiaUnits=kg*m^2  ProductsOfInertia=[0 0 0]  ProductsOfInertiaUnits=kg*m^2  DensityBased=on  Density=DensityTube  DensityUnits=kg/(m^3)  DoExposeReferenceFrame=on  SerializedFrames=<Frames/>  GraphicType=FromGeometry  MarkerShape=Sphere  MarkerSize=10  MarkerSizeUnits=m  GraphicVisPropType=SimpleVisualProperties  GraphicDiffuseColor=[0.5 0.5 0.5]  GraphicSpecularColor=[0.5 0.5 0.5 1.0]  GraphicAmbientColor=[0.15 0.15 0.15 1.0]  GraphicEmissiveColor=[0.0 0.0 0.0 1.0]  GraphicShininess=75  GraphicOpacity=1.0  GeometryShape=Sphere  RectangleSize=[1 1]  RectangleSizeUnits=m  BrickDimensions=[1 1 1]  BrickDimensionUnits=m  CylinderRadius=RadiusTube  CylinderRadiusUnits=m  CylinderLength=RodLength  CylinderLengthUnits=m  SphereRadius=.5  SphereRadiusUnits=m  EllipsoidRadii=[1 1 1]  EllipsoidRadiiUnits=m  ExtrusionCrossSection=[1 1; -1 1; -1 -1; 1 -1]  ExtrusionCrossSectionUnits=m  ExtrusionLength=1  ExtrusionLengthUnits=m  PolygonNumSides=3  PolygonOuterRadius=1  PolygonOuterRadiusUnits=m  ExtGeomFileType=STL  ExtGeomFileUnits=m  RevolutionCrossSection=[1 1; 1 -1; 2 -1; 2 1]  RevolutionCrossSectionUnits=m  RevolutionExtent=Full  RevolutionAngle=180  RevolutionAngleUnits=deg  BlockFunction=simmechanics.library.body_elements.solid
  HorizontalBar3 : sm_lib/Body Elements/Solid  InertiaType=PointMass  Mass=462.5  MassUnits=kg  CenterOfMass=[0 0 0]  CenterOfMassUnits=m  MomentsOfInertia=[1 1 1]  MomentsOfInertiaUnits=kg*m^2  ProductsOfInertia=[0 0 0]  ProductsOfInertiaUnits=kg*m^2  DensityBased=on  Density=DensityTube  DensityUnits=kg/(m^3)  DoExposeReferenceFrame=on  SerializedFrames=<Frames/>  GraphicType=FromGeometry  MarkerShape=Sphere  MarkerSize=10  MarkerSizeUnits=m  GraphicVisPropType=SimpleVisualProperties  GraphicDiffuseColor=[0.5 0.5 0.5]  GraphicSpecularColor=[0.5 0.5 0.5 1.0]  GraphicAmbientColor=[0.15 0.15 0.15 1.0]  GraphicEmissiveColor=[0.0 0.0 0.0 1.0]  GraphicShininess=75  GraphicOpacity=1.0  GeometryShape=Sphere  RectangleSize=[1 1]  RectangleSizeUnits=m  BrickDimensions=[1 1 1]  BrickDimensionUnits=m  CylinderRadius=RadiusTube  CylinderRadiusUnits=m  CylinderLength=RodLength  CylinderLengthUnits=m  SphereRadius=.5  SphereRadiusUnits=m  EllipsoidRadii=[1 1 1]  EllipsoidRadiiUnits=m  ExtrusionCrossSection=[1 1; -1 1; -1 -1; 1 -1]  ExtrusionCrossSectionUnits=m  ExtrusionLength=1  ExtrusionLengthUnits=m  PolygonNumSides=3  PolygonOuterRadius=1  PolygonOuterRadiusUnits=m  ExtGeomFileType=STL  ExtGeomFileUnits=m  RevolutionCrossSection=[1 1; 1 -1; 2 -1; 2 1]  RevolutionCrossSectionUnits=m  RevolutionExtent=Full  RevolutionAngle=180  RevolutionAngleUnits=deg  BlockFunction=simmechanics.library.body_elements.solid
  Motor Clockwise 3 : Library_Octocopter/Motor Clockwise1
  Motor Counter Clockwise 8 : Library_Octocopter/Motor Counter Clockwise1
  Rigid Transform1 : sm_lib/Frames and Transforms/Rigid Transform  TranslationMethod=Cartesian  TranslationLengthUnit=m  TranslationStandardAxis=+Z  TranslationStandardOffset=0  TranslationCartesianOffset=HorizontalBar1  TranslationROffset=0  TranslationROffsetUnits=m  TranslationZOffset=0  TranslationZOffsetUnits=m  TranslationThetaOffset=0  TranslationThetaOffsetUnits=deg  RotationMethod=None  RotationAngleUnits=deg  RotationStandardAxis=+Z  RotationAngle=0  RotationArbitraryAxis=[0 0 1]  FollAlignAxisA=+X  BaseAlignAxisA=+Y  FollAlignAxisB=+Y  BaseAlignAxisB=+Z  RotationSequenceAxes=FollowerAxes  RotationSequence=XYX  RotationSequenceAngles=[0 0 0]  RotationSequenceAnglesUnits=deg  RotationMatrix=[1 0 0; 0 1 0; 0 0 1]  BlockFunction=simmechanics.library.frames_transforms.rigid_transform
  Rigid Transform2 : sm_lib/Frames and Transforms/Rigid Transform  TranslationMethod=Cartesian  TranslationLengthUnit=m  TranslationStandardAxis=+Z  TranslationStandardOffset=0  TranslationCartesianOffset=PositionEngine8  TranslationROffset=0  TranslationROffsetUnits=m  TranslationZOffset=0  TranslationZOffsetUnits=m  TranslationThetaOffset=0  TranslationThetaOffsetUnits=deg  RotationMethod=None  RotationAngleUnits=deg  RotationStandardAxis=+Z  RotationAngle=0  RotationArbitraryAxis=[0 0 1]  FollAlignAxisA=+X  BaseAlignAxisA=+Y  FollAlignAxisB=+Y  BaseAlignAxisB=+Z  RotationSequenceAxes=FollowerAxes  RotationSequence=XYX  RotationSequenceAngles=[0 0 0]  RotationSequenceAnglesUnits=deg  RotationMatrix=[1 0 0; 0 1 0; 0 0 1]  BlockFunction=simmechanics.library.frames_transforms.rigid_transform
  Rigid Transform3 : sm_lib/Frames and Transforms/Rigid Transform  TranslationMethod=Cartesian  TranslationLengthUnit=m  TranslationStandardAxis=+Z  TranslationStandardOffset=0  TranslationCartesianOffset=[0 0 0]  TranslationROffset=0  TranslationROffsetUnits=m  TranslationZOffset=0  TranslationZOffsetUnits=m  TranslationThetaOffset=0  TranslationThetaOffsetUnits=deg  RotationMethod=StandardAxis  RotationAngleUnits=deg  RotationStandardAxis=+Y  RotationAngle=90  RotationArbitraryAxis=[0 0 1]  FollAlignAxisA=+X  BaseAlignAxisA=+Y  FollAlignAxisB=+Y  BaseAlignAxisB=+Z  RotationSequenceAxes=FollowerAxes  RotationSequence=XYX  RotationSequenceAngles=[0 0 0]  RotationSequenceAnglesUnits=deg  RotationMatrix=[1 0 0; 0 1 0; 0 0 1]  BlockFunction=simmechanics.library.frames_transforms.rigid_transform
  Rigid Transform6 : sm_lib/Frames and Transforms/Rigid Transform  TranslationMethod=Cartesian  TranslationLengthUnit=m  TranslationStandardAxis=+Z  TranslationStandardOffset=0  TranslationCartesianOffset=PositionEngine3  TranslationROffset=0  TranslationROffsetUnits=m  TranslationZOffset=0  TranslationZOffsetUnits=m  TranslationThetaOffset=0  TranslationThetaOffsetUnits=deg  RotationMethod=None  RotationAngleUnits=deg  RotationStandardAxis=+Z  RotationAngle=0  RotationArbitraryAxis=[0 0 1]  FollAlignAxisA=+X  BaseAlignAxisA=+Y  FollAlignAxisB=+Y  BaseAlignAxisB=+Z  RotationSequenceAxes=FollowerAxes  RotationSequence=XYX  RotationSequenceAngles=[0 0 0]  RotationSequenceAnglesUnits=deg  RotationMatrix=[1 0 0; 0 1 0; 0 0 1]  BlockFunction=simmechanics.library.frames_transforms.rigid_transform
  Step : Step  Time=75
  Step1 : Step  Time=75
  Switch : Switch  Criteria=u2 > Threshold  Threshold=0.5
  Switch1 : Switch  Criteria=u2 > Threshold  Threshold=0.5
  Conn1 : PMIOPort  Port=1  Side=Right
  wires:
  Switch/1 -> Motor Clockwise 3/1
  Motor 3 cw/1 -> Switch/3
  Constant/1 -> Switch/1
  Switch1/1 -> Motor Counter Clockwise 8/1
  Motor 8 ccw/1 -> Switch1/3
  Constant1/1 -> Switch1/1
  connections:
  Rigid Transform1/LConn1 -- Rigid Transform6/LConn1 -- Rigid Transform2/LConn1 -- Conn1/RConn1
  HorizontalBar1/RConn1 -- Rigid Transform3/RConn1
  Rigid Transform2/RConn1 -- HorizontalBar2/RConn1 -- Motor Counter Clockwise 8/RConn1
  Rigid Transform3/LConn1 -- Rigid Transform1/RConn1
  Motor Clockwise 3/RConn1 -- HorizontalBar3/RConn1 -- Rigid Transform6/RConn1

== system DuoCopter1AGRESSIVE/Octocopter/Horizontal 2 ==
  Motor 7 cw : Inport
  Motor 4 ccw : Inport  Port=2
  Constant : Constant  Value=0
  HorizontalBar1 : sm_lib/Body Elements/Solid  InertiaType=PointMass  Mass=462.5  MassUnits=kg  CenterOfMass=[0 0 0]  CenterOfMassUnits=m  MomentsOfInertia=[1 1 1]  MomentsOfInertiaUnits=kg*m^2  ProductsOfInertia=[0 0 0]  ProductsOfInertiaUnits=kg*m^2  DensityBased=on  Density=DensityTube  DensityUnits=kg/(m^3)  DoExposeReferenceFrame=on  SerializedFrames=<Frames/>  GraphicType=FromGeometry  MarkerShape=Sphere  MarkerSize=10  MarkerSizeUnits=m  GraphicVisPropType=SimpleVisualProperties  GraphicDiffuseColor=[0.5 0.5 0.5]  GraphicSpecularColor=[0.5 0.5 0.5 1.0]  GraphicAmbientColor=[0.15 0.15 0.15 1.0]  GraphicEmissiveColor=[0.0 0.0 0.0 1.0]  GraphicShininess=75  GraphicOpacity=1.0  GeometryShape=Sphere  RectangleSize=[1 1]  RectangleSizeUnits=m  BrickDimensions=[1 1 1]  BrickDimensionUnits=m  CylinderRadius=RadiusTube  CylinderRadiusUnits=m  CylinderLength=RodLength  CylinderLengthUnits=m  SphereRadius=.5  SphereRadiusUnits=m  EllipsoidRadii=[1 1 1]  EllipsoidRadiiUnits=m  ExtrusionCrossSection=[1 1; -1 1; -1 -1; 1 -1]  ExtrusionCrossSectionUnits=m  ExtrusionLength=1  ExtrusionLengthUnits=m  PolygonNumSides=3  PolygonOuterRadius=1  PolygonOuterRadiusUnits=m  ExtGeomFileType=STL  ExtGeomFileUnits=m  RevolutionCrossSection=[1 1; 1 -1; 2 -1; 2 1]  RevolutionCrossSectionUnits=m  RevolutionExtent=Full  RevolutionAngle=180  RevolutionAngleUnits=deg  BlockFunction=simmechanics.library.body_elements.solid
  HorizontalBar2 : sm_lib/Body Elements/Solid  InertiaType=CalculateFromGeometry  Mass=RodMass  MassUnits=kg  CenterOfMass=[0 0 0]  CenterOfMassUnits=m  MomentsOfInertia=[1 1 1]  MomentsOfInertiaUnits=kg*m^2  ProductsOfInertia=[0 0 0]  ProductsOfInertiaUnits=kg*m^2  DensityBased=off  Density=DensityTube  DensityUnits=kg/(m^3)  DoExposeReferenceFrame=on  SerializedFrames=<Frames/>  GraphicType=FromGeometry  MarkerShape=Sphere  MarkerSize=10  MarkerSizeUnits=m  GraphicVisPropType=SimpleVisualProperties  GraphicDiffuseColor=[0.5 0.5 0.5]  GraphicSpecularColor=[0.5 0.5 0.5 1.0]  GraphicAmbientColor=[0.15 0.15 0.15 1.0]  GraphicEmissiveColor=[0.0 0.0 0.0 1.0]  GraphicShininess=75  GraphicOpacity=1.0  GeometryShape=Cylinder  RectangleSize=[1 1]  RectangleSizeUnits=m  BrickDimensions=[1 1 1]  BrickDimensionUnits=m  CylinderRadius=RadiusTube  CylinderRadiusUnits=m  CylinderLength=RodLength  CylinderLengthUnits=m  SphereRadius=1  SphereRadiusUnits=m  EllipsoidRadii=[1 1 1]  EllipsoidRadiiUnits=m  ExtrusionCrossSection=[1 1; -1 1; -1 -1; 1 -1]  ExtrusionCrossSectionUnits=m  ExtrusionLength=1  ExtrusionLengthUnits=m  PolygonNumSides=3  PolygonOuterRadius=1  PolygonOuterRadiusUnits=m  ExtGeomFileType=STL  ExtGeomFileUnits=m  RevolutionCrossSection=[1 1; 1 -1; 2 -1; 2 1]  RevolutionCrossSectionUnits=m  RevolutionExtent=Full  RevolutionAngle=180  RevolutionAngleUnits=deg  BlockFunction=simmechanics.library.body_elements.solid
  HorizontalBar3 : sm_lib/Body Elements/Solid  InertiaType=PointMass  Mass=462.5  MassUnits=kg  CenterOfMass=[0 0 0]  CenterOfMassUnits=m  MomentsOfInertia=[1 1 1]  MomentsOfInertiaUnits=kg*m^2  ProductsOfInertia=[0 0 0]  ProductsOfInertiaUnits=kg*m^2  DensityBased=on  Density=DensityTube  DensityUnits=kg/(m^3)  DoExposeReferenceFrame=on  SerializedFrames=<Frames/>  GraphicType=FromGeometry  MarkerShape=Sphere  MarkerSize=10  MarkerSizeUnits=m  GraphicVisPropType=SimpleVisualProperties  GraphicDiffuseColor=[0.5 0.5 0.5]  GraphicSpecularColor=[0.5 0.5 0.5 1.0]  GraphicAmbientColor=[0.15 0.15 0.15 1.0]  GraphicEmissiveColor=[0.0 0.0 0.0 1.0]  GraphicShininess=75  GraphicOpacity=1.0  GeometryShape=Sphere  RectangleSize=[1 1]  RectangleSizeUnits=m  BrickDimensions=[1 1 1]  BrickDimensionUnits=m  CylinderRadius=RadiusTube  CylinderRadiusUnits=m  CylinderLength=RodLength  CylinderLengthUnits=m  SphereRadius=.5  SphereRadiusUnits=m  EllipsoidRadii=[1 1 1]  EllipsoidRadiiUnits=m  ExtrusionCrossSection=[1 1; -1 1; -1 -1; 1 -1]  ExtrusionCrossSectionUnits=m  ExtrusionLength=1  ExtrusionLengthUnits=m  PolygonNumSides=3  PolygonOuterRadius=1  PolygonOuterRadiusUnits=m  ExtGeomFileType=STL  ExtGeomFileUnits=m  RevolutionCrossSection=[1 1; 1 -1; 2 -1; 2 1]  RevolutionCrossSectionUnits=m  RevolutionExtent=Full  RevolutionAngle=180  RevolutionAngleUnits=deg  BlockFunction=simmechanics.library.body_elements.solid
  Motor Clockwise 7 : Library_Octocopter/Motor Clockwise1
  Motor Counter Clockwise 4 : Library_Octocopter/Motor Counter Clockwise1
  Rigid Transform4 : sm_lib/Frames and Transforms/Rigid Transform  TranslationMethod=Cartesian  TranslationLengthUnit=m  TranslationStandardAxis=+Z  TranslationStandardOffset=0  TranslationCartesianOffset=HorizontalBar2  TranslationROffset=0  TranslationROffsetUnits=m  TranslationZOffset=0  TranslationZOffsetUnits=m  TranslationThetaOffset=0  TranslationThetaOffsetUnits=deg  RotationMethod=None  RotationAngleUnits=deg  RotationStandardAxis=+Z  RotationAngle=0  RotationArbitraryAxis=[0 0 1]  FollAlignAxisA=+X  BaseAlignAxisA=+Y  FollAlignAxisB=+Y  BaseAlignAxisB=+Z  RotationSequenceAxes=FollowerAxes  RotationSequence=XYX  RotationSequenceAngles=[0 0 0]  RotationSequenceAnglesUnits=deg  RotationMatrix=[1 0 0; 0 1 0; 0 0 1]  BlockFunction=simmechanics.library.frames_transforms.rigid_transform
  Rigid Transform5 : sm_lib/Frames and Transforms/Rigid Transform  TranslationMethod=Cartesian  TranslationLengthUnit=m  TranslationStandardAxis=+Z  TranslationStandardOffset=0  TranslationCartesianOffset=PositionEngine7  TranslationROffset=0  TranslationROffsetUnits=m  TranslationZOffset=0  TranslationZOffsetUnits=m  TranslationThetaOffset=0  TranslationThetaOffsetUnits=deg  RotationMethod=None  RotationAngleUnits=deg  RotationStandardAxis=+Z  RotationAngle=0  RotationArbitraryAxis=[0 0 1]  FollAlignAxisA=+X  BaseAlignAxisA=+Y  FollAlignAxisB=+Y  BaseAlignAxisB=+Z  RotationSequenceAxes=FollowerAxes  RotationSequence=XYX  RotationSequenceAngles=[0 0 0]  RotationSequenceAnglesUnits=deg  RotationMatrix=[1 0 0; 0 1 0; 0 0 1]  BlockFunction=simmechanics.library.frames_transforms.rigid_transform
  Rigid Transform7 : sm_lib/Frames and Transforms/Rigid Transform  TranslationMethod=Cartesian  TranslationLengthUnit=m  TranslationStandardAxis=+Z  TranslationStandardOffset=0  TranslationCartesianOffset=[0 0 0]  TranslationROffset=0  TranslationROffsetUnits=m  TranslationZOffset=0  TranslationZOffsetUnits=m  TranslationThetaOffset=0  TranslationThetaOffsetUnits=deg  RotationMethod=StandardAxis  RotationAngleUnits=deg  RotationStandardAxis=+Y  RotationAngle=90  RotationArbitraryAxis=[0 0 1]  FollAlignAxisA=+X  BaseAlignAxisA=+Y  FollAlignAxisB=+Y  BaseAlignAxisB=+Z  RotationSequenceAxes=FollowerAxes  RotationSequence=XYX  RotationSequenceAngles=[0 0 0]  RotationSequenceAnglesUnits=deg  RotationMatrix=[1 0 0; 0 1 0; 0 0 1]  BlockFunction=simmechanics.library.frames_transforms.rigid_transform
  Rigid Transform8 : sm_lib/Frames and Transforms/Rigid Transform  TranslationMethod=Cartesian  TranslationLengthUnit=m  TranslationStandardAxis=+Z  TranslationStandardOffset=0  TranslationCartesianOffset=PositionEngine4  TranslationROffset=0  TranslationROffsetUnits=m  TranslationZOffset=0  TranslationZOffsetUnits=m  TranslationThetaOffset=0  TranslationThetaOffsetUnits=deg  RotationMethod=None  RotationAngleUnits=deg  RotationStandardAxis=+Z  RotationAngle=0  RotationArbitraryAxis=[0 0 1]  FollAlignAxisA=+X  BaseAlignAxisA=+Y  FollAlignAxisB=+Y  BaseAlignAxisB=+Z  RotationSequenceAxes=FollowerAxes  RotationSequence=XYX  RotationSequenceAngles=[0 0 0]  RotationSequenceAnglesUnits=deg  RotationMatrix=[1 0 0; 0 1 0; 0 0 1]  BlockFunction=simmechanics.library.frames_transforms.rigid_transform
  Step : Step  Time=72
  Switch : Switch  Criteria=u2 > Threshold  Threshold=0.5
  Conn1 : PMIOPort  Port=1  Side=Right
  wires:
  Motor 4 ccw/1 -> Motor Counter Clockwise 4/1
  Switch/1 -> Motor Clockwise 7/1
  Motor 7 cw/1 -> Switch/3
  Constant/1 -> Switch/1
  Step/1 -> Switch/2
  connections:
  Rigid Transform7/LConn1 -- Rigid Transform4/RConn1
  Motor Clockwise 7/RConn1 -- HorizontalBar1/RConn1 -- Rigid Transform5/RConn1
  HorizontalBar2/RConn1 -- Rigid Transform7/RConn1
  Rigid Transform8/LConn1 -- Conn1/RConn1 -- Rigid Transform4/LConn1 -- Rigid Transform5/LConn1
  Motor Counter Clockwise 4/RConn1 -- HorizontalBar3/RConn1 -- Rigid Transform8/RConn1
